simulink model "MR_CIGRE_CONVENCIONAL"  (R2017b)
settings: Solver=ode23tb  StartTime=0.0  StopTime=t_sim  RelTol=1e-4
values from neighbouring files (symbols this model uses):
  BAT1_CONT = 0    [Dados_MR_CIGRE_convencional.m]
  BAT2_CONT = 0    [Dados_MR_CIGRE_convencional.m]
  cont_fre = 1    [Dados_de_Sec.m]
  cont_ten = 1    [Dados_de_Sec.m]
  f0 = 50    [Dados_MR_CIGRE_convencional.m]
  Kie = 10    [Dados_de_Sec.m]
  Kiw = 2.5    [Dados_de_Sec.m]
  Kpe = 0.1    [Dados_de_Sec.m]
  Kpw = 0.23    [Dados_de_Sec.m]
  P_Solar1 = 21e3    (= 21000)    [Dados_MR_CIGRE_convencional.m]
  P_Solar2 = 21e3    (= 21000)    [Dados_MR_CIGRE_convencional.m]
  PQ_ref_time_bat1 = t_estab    (= 1)    [Dados_MR_CIGRE_convencional.m]
  Pref_Bat1 = 0*1e3    (= 0)    [Dados_MR_CIGRE_convencional.m]
  Qref_Bat1 = 0*1e3    (= 0)    [Dados_MR_CIGRE_convencional.m]
  Qref_Solar = 0    [Automatico_XXX.m]    (also in Dados_MR_CIGRE_convencional.m)
  Sb_Bat1 = 45e3    (= 45000)    [Dados_MR_CIGRE_convencional.m]
  Sb_sol1 = 20e3    (= 20000)    [Dados_MR_CIGRE_convencional.m]
  Sb_sol2 = 20e3    (= 20000)    [Dados_MR_CIGRE_convencional.m]
  t_atraso = 0    [Dados_MR_CIGRE_convencional.m]
  TDR1 = 80    [Dados_de_Cargas.m]
  TDR11 = 80    [Dados_de_Cargas.m]
  TDR15 = 80    [Dados_de_Cargas.m]
  TDR16 = 80    [Dados_de_Cargas.m]
  TDR17 = 80    [Dados_de_Cargas.m]
  TDR18 = 80    [Dados_de_Cargas.m]
  tilha = 0.6    [Dados_MR_CIGRE_convencional.m]
  TLR11 = 60    [Dados_de_Cargas.m]
  TLR15 = 3.5    [Dados_de_Cargas.m]
  TLR16 = 6    [Dados_de_Cargas.m]
  TLR17 = 60    [Dados_de_Cargas.m]
  TLR18 = 60    [Dados_de_Cargas.m]
  tsinc = 6    [Dados_MR_CIGRE_convencional.m]
  vref1 = 1    [Dados_de_Sec.m]
  Vref_sec = 1    [Dados_de_Sec.m]
  Vs1 = 20000    [Dados_MR_CIGRE_convencional.m]
  Vs2 = 400    [Dados_MR_CIGRE_convencional.m]
  w0 = 2*pi*f0    (= 314.159265359)    [Dados_MR_CIGRE_convencional.m]
  wref_sec = 1    [Dados_de_Sec.m]
undefined symbols (not defined in the file or in its folder): Cdc, Cdc_Bat1, Cf, Cf_Bat1, I_max_Bat1, Imax_solar1, Imax_solar2, Is_bat1, K_iff_Bat1, Kcij, Ki_Bat1, Ki_interm, Kp_Bat1, Kp_cp, Kp_cr, Kp_interm, Kv_Bat1, Kvi_DC, Kvp_DC, L, L_10_18, L_12_13, L_13_14, L_14_15, L_1_2, L_2_3, L_3_11, L_3_4, L_4_12, L_4_5, L_5_6, L_6_16, L_6_7, L_7_8, L_8_9, L_9_10, L_9_17, L_Bat1, L_Bat2, L_Virt_Bat1, L_Virt_Bat2, LC_Bat2, Lfsj, LPF_Ci_Bat1, LPF_Ci_Bat2, LPF_Cv_Bat1, LPF_P_Bat1, LPF_P_Interm, LPF_Q_Bat1, LPF_Vdc, m_Bat1, n_Bat1, PQ_ref_taxavar_bat1, R, R_10_18, R_12_13, R_13_14, R_14_15, R_1_2, R_2_3 ... (+27)
libraries: powerlib x158, powerlib_meascontrol x59, re_lib x2, simulink x1
(part 2 of 4)

== system MR_CIGRE_CONVENCIONAL/R11 ==
  1/Ib : Gain  Gain=(1)/(sqrt(2))
  1/Vb : Gain  Gain=sqrt(3)/(1*sqrt(2))
  BCarga : powerlib/Measurements/Three-Phase V-I Measurement  VoltageMeasurement=phase-to-ground  SetLabelV=off  LabelV=Vabc_B2  Vpu=off  VpuLL=off  CurrentMeasurement=yes  SetLabelI=off  LabelI=Iabc_B120  Ipu=off  Pbase=100e6  Vbase=Vs2  OutputType=Complex  PhasorSimulation=on  PSBequivalent=0
  CCV1 : powerlib/Elements/Three-Phase Breaker  InitialState=open  SwitchA=on  SwitchB=on  SwitchC=on  SwitchTimes=[TLR11 TDR11]  External=off  BreakerResistance=0.01  SnubberResistance=1e5  SnubberCapacitance=inf  Measurements=None
      settings: AttributesFormatString=\n
  Carga Fixa : powerlib/Elements/Three-Phase Series RLC Load  LConnTagsString=A|B|C  Configuration=Y (grounded)  NominalVoltage=Vs2  Vabc=[1e3 1e3 1e3]  Vabcp=[1e3 1e3 1e3]  NominalFrequency=f0  UnbalancedPower=off  ActivePower=PLoadR11  InductivePower=QLoadR11  CapacitivePower=0  Pabc=[10e3 9e3 11e3]  QLabc=[100 90 110]  QCabc=[100 90 110]  Pabcp=[10e3 9e3 11e3]  QLabcp=[100 90 110]  QCabcp=[100 90 110]  Measurements=None  LoadType=constant Z
  Carga Variável : powerlib/Elements/Three-Phase Series RLC Load  LConnTagsString=A|B|C  Configuration=Y (grounded)  NominalVoltage=Vs2  Vabc=[1e3 1e3 1e3]  Vabcp=[1e3 1e3 1e3]  NominalFrequency=f0  UnbalancedPower=off  ActivePower=P_var_loadR11  InductivePower=Q_var_loadR11  CapacitivePower=0  Pabc=[10e3 9e3 11e3]  QLabc=[100 90 110]  QCabc=[100 90 110]  Pabcp=[10e3 9e3 11e3]  QLabcp=[100 90 110]  QCabcp=[100 90 110]  Measurements=None  LoadType=constant Z
  Dados_C1 : ToWorkspace  VariableName=R11  SaveFormat=Structure With Time  SampleTime=-1
  Ip : powerlib_meascontrol/Measurements/Sequence Analyzer  Freq=f0  n=1  seq=Positive  InInit=[1, 0]  Ts=0
      settings: SourceProductName=Simscape Power Systems  SourceProductBaseCode=PS
  Mux9 : Mux
  Power : powerlib_meascontrol/Measurements/Power (Positive-Sequence)  Freq=f0  Vinit=[0, 0]  Iinit=[0, 0]  Ts=0
      settings: SourceProductName=Simscape Power Systems  SourceProductBaseCode=PS
  Reshape : Reshape  OutputDimensions=[1,7]
  Vp : powerlib_meascontrol/Measurements/Sequence Analyzer  Freq=f0  n=1  seq=Positive  InInit=[1, 0]  Ts=0
      settings: SourceProductName=Simscape Power Systems  SourceProductBaseCode=PS
  fa : PMIOPort  Port=1  Side=Left
  fb : PMIOPort  Port=2  Side=Left
  fc : PMIOPort  Port=3  Side=Left
  P : Outport
  V : Outport  Port=2
  Q : Outport  Port=3
  I : Outport  Port=4
  wires:
  BCarga/1 -> Power/1, Vp/1
  Mux9/1 -> Reshape/1
  BCarga/2 -> Power/2, Ip/1
  Power/1 -> Mux9/1, P/1
  1/Vb/1 -> V/1, Mux9/2
  1/Ib/1 -> I/1, Mux9/4
  Vp/1 -> 1/Vb/1
  Ip/1 -> 1/Ib/1
  Power/2 -> Q/1, Mux9/3
  Reshape/1 -> Dados_C1/1
  connections:
  BCarga/LConn3 -- fc/RConn1
  BCarga/LConn2 -- fb/RConn1
  BCarga/LConn1 -- fa/RConn1
  BCarga/RConn3 -- CCV1/RConn3 -- Carga Fixa/LConn3
  BCarga/RConn1 -- CCV1/RConn1 -- Carga Fixa/LConn1
  BCarga/RConn2 -- CCV1/RConn2 -- Carga Fixa/LConn2
  CCV1/LConn1 -- Carga Variável/LConn1
  CCV1/LConn3 -- Carga Variável/LConn3
  CCV1/LConn2 -- Carga Variável/LConn2

== system MR_CIGRE_CONVENCIONAL/R12_R13 ==
  1 : powerlib/Elements/Series RLC Branch  LConnTagsString=__new0  RConnTagsString=__new0  BranchType=RL  Resistance=R_12_13  Inductance=L_12_13  SetiL0=off  InitialCurrent=0  Capacitance=1e-6  Setx0=off  InitialVoltage=0  Measurements=None
  2 : powerlib/Elements/Series RLC Branch  LConnTagsString=__new0  RConnTagsString=__new0  BranchType=RL  Resistance=R_12_13  Inductance=L_12_13  SetiL0=off  InitialCurrent=0  Capacitance=1e-6  Setx0=off  InitialVoltage=0  Measurements=None
  3 : powerlib/Elements/Series RLC Branch  LConnTagsString=__new0  RConnTagsString=__new0  BranchType=RL  Resistance=R_12_13  Inductance=L_12_13  SetiL0=off  InitialCurrent=0  Capacitance=1e-6  Setx0=off  InitialVoltage=0  Measurements=None
  A : PMIOPort  Port=1  Side=Left
  a : PMIOPort  Port=2  Side=Right
  B : PMIOPort  Port=3  Side=Left
  b : PMIOPort  Port=4  Side=Right
  C : PMIOPort  Port=5  Side=Left
  c : PMIOPort  Port=6  Side=Right
  connections:
  1/LConn1 -- A/RConn1
  2/LConn1 -- B/RConn1
  3/LConn1 -- C/RConn1
  1/RConn1 -- a/RConn1
  2/RConn1 -- b/RConn1
  3/RConn1 -- c/RConn1

== system MR_CIGRE_CONVENCIONAL/R13_R14 ==
  1 : powerlib/Elements/Series RLC Branch  LConnTagsString=__new0  RConnTagsString=__new0  BranchType=RL  Resistance=R_13_14  Inductance=L_13_14  SetiL0=off  InitialCurrent=0  Capacitance=1e-6  Setx0=off  InitialVoltage=0  Measurements=None
  2 : powerlib/Elements/Series RLC Branch  LConnTagsString=__new0  RConnTagsString=__new0  BranchType=RL  Resistance=R_13_14  Inductance=L_13_14  SetiL0=off  InitialCurrent=0  Capacitance=1e-6  Setx0=off  InitialVoltage=0  Measurements=None
  3 : powerlib/Elements/Series RLC Branch  LConnTagsString=__new0  RConnTagsString=__new0  BranchType=RL  Resistance=R_13_14  Inductance=L_13_14  SetiL0=off  InitialCurrent=0  Capacitance=1e-6  Setx0=off  InitialVoltage=0  Measurements=None
  A : PMIOPort  Port=1  Side=Left
  a : PMIOPort  Port=2  Side=Right
  B : PMIOPort  Port=3  Side=Left
  b : PMIOPort  Port=4  Side=Right
  C : PMIOPort  Port=5  Side=Left
  c : PMIOPort  Port=6  Side=Right
  connections:
  1/LConn1 -- A/RConn1
  2/LConn1 -- B/RConn1
  3/LConn1 -- C/RConn1
  1/RConn1 -- a/RConn1
  2/RConn1 -- b/RConn1
  3/RConn1 -- c/RConn1

== system MR_CIGRE_CONVENCIONAL/R14_R15 ==
  1 : powerlib/Elements/Series RLC Branch  LConnTagsString=__new0  RConnTagsString=__new0  BranchType=RL  Resistance=R_14_15  Inductance=L_14_15  SetiL0=off  InitialCurrent=0  Capacitance=1e-6  Setx0=off  InitialVoltage=0  Measurements=None
  2 : powerlib/Elements/Series RLC Branch  LConnTagsString=__new0  RConnTagsString=__new0  BranchType=RL  Resistance=R_14_15  Inductance=L_14_15  SetiL0=off  InitialCurrent=0  Capacitance=1e-6  Setx0=off  InitialVoltage=0  Measurements=None
  3 : powerlib/Elements/Series RLC Branch  LConnTagsString=__new0  RConnTagsString=__new0  BranchType=RL  Resistance=R_14_15  Inductance=L_14_15  SetiL0=off  InitialCurrent=0  Capacitance=1e-6  Setx0=off  InitialVoltage=0  Measurements=None
  A : PMIOPort  Port=1  Side=Left
  a : PMIOPort  Port=2  Side=Right
  B : PMIOPort  Port=3  Side=Left
  b : PMIOPort  Port=4  Side=Right
  C : PMIOPort  Port=5  Side=Left
  c : PMIOPort  Port=6  Side=Right
  connections:
  1/LConn1 -- A/RConn1
  2/LConn1 -- B/RConn1
  3/LConn1 -- C/RConn1
  1/RConn1 -- a/RConn1
  2/RConn1 -- b/RConn1
  3/RConn1 -- c/RConn1

== system MR_CIGRE_CONVENCIONAL/R15 ==
  1/Ib : Gain  Gain=(1)/(sqrt(2))
  1/Vb : Gain  Gain=sqrt(3)/(1*sqrt(2))
  BCarga : powerlib/Measurements/Three-Phase V-I Measurement  VoltageMeasurement=phase-to-ground  SetLabelV=off  LabelV=Vabc_B2  Vpu=off  VpuLL=off  CurrentMeasurement=yes  SetLabelI=off  LabelI=Iabc_B120  Ipu=off  Pbase=100e6  Vbase=Vs2  OutputType=Complex  PhasorSimulation=on  PSBequivalent=0
  CCV : powerlib/Elements/Three-Phase Breaker  InitialState=open  SwitchA=on  SwitchB=on  SwitchC=on  SwitchTimes=[TLR15 TDR15]  External=off  BreakerResistance=0.01  SnubberResistance=1e5  SnubberCapacitance=inf  Measurements=None
      settings: AttributesFormatString=\n
  Carga Fixa : powerlib/Elements/Three-Phase Series RLC Load  LConnTagsString=A|B|C  Configuration=Y (grounded)  NominalVoltage=Vs2  Vabc=[1e3 1e3 1e3]  Vabcp=[1e3 1e3 1e3]  NominalFrequency=f0  UnbalancedPower=off  ActivePower=PLoadR15  InductivePower=QLoadR15  CapacitivePower=0  Pabc=[10e3 9e3 11e3]  QLabc=[100 90 110]  QCabc=[100 90 110]  Pabcp=[10e3 9e3 11e3]  QLabcp=[100 90 110]  QCabcp=[100 90 110]  Measurements=None  LoadType=constant Z
  Carga Variável : powerlib/Elements/Three-Phase Series RLC Load  LConnTagsString=A|B|C  Configuration=Y (grounded)  NominalVoltage=Vs2  Vabc=[1e3 1e3 1e3]  Vabcp=[1e3 1e3 1e3]  NominalFrequency=f0  UnbalancedPower=off  ActivePower=P_var_loadR15  InductivePower=Q_var_loadR15  CapacitivePower=0  Pabc=[10e3 9e3 11e3]  QLabc=[100 90 110]  QCabc=[100 90 110]  Pabcp=[10e3 9e3 11e3]  QLabcp=[100 90 110]  QCabcp=[100 90 110]  Measurements=None  LoadType=constant Z
  Dados_C1 : ToWorkspace  VariableName=R15  SaveFormat=Structure With Time  SampleTime=-1
  Ip : powerlib_meascontrol/Measurements/Sequence Analyzer  Freq=f0  n=1  seq=Positive  InInit=[1, 0]  Ts=0
      settings: SourceProductName=Simscape Power Systems  SourceProductBaseCode=PS
  Mux9 : Mux
  Power : powerlib_meascontrol/Measurements/Power (Positive-Sequence)  Freq=f0  Vinit=[0, 0]  Iinit=[0, 0]  Ts=0
      settings: SourceProductName=Simscape Power Systems  SourceProductBaseCode=PS
  Reshape : Reshape  OutputDimensions=[1,7]
  Vp : powerlib_meascontrol/Measurements/Sequence Analyzer  Freq=f0  n=1  seq=Positive  InInit=[1, 0]  Ts=0
      settings: SourceProductName=Simscape Power Systems  SourceProductBaseCode=PS
  fa : PMIOPort  Port=1  Side=Left
  fb : PMIOPort  Port=2  Side=Left
  fc : PMIOPort  Port=3  Side=Left
  P : Outport
  V : Outport  Port=2
  Q : Outport  Port=3
  I : Outport  Port=4
  wires:
  Mux9/1 -> Reshape/1
  BCarga/2 -> Power/2, Ip/1
  1/Ib/1 -> I/1, Mux9/4
  Ip/1 -> 1/Ib/1
  1/Vb/1 -> V/1, Mux9/2
  Vp/1 -> 1/Vb/1
  BCarga/1 -> Power/1, Vp/1
  Power/2 -> Q/1, Mux9/3
  Power/1 -> Mux9/1, P/1
  Reshape/1 -> Dados_C1/1
  connections:
  BCarga/LConn3 -- fc/RConn1
  BCarga/LConn2 -- fb/RConn1
  BCarga/LConn1 -- fa/RConn1
  BCarga/RConn3 -- Carga Fixa/LConn3 -- CCV/RConn3
  BCarga/RConn1 -- Carga Fixa/LConn1 -- CCV/RConn1
  BCarga/RConn2 -- Carga Fixa/LConn2 -- CCV/RConn2
  CCV/LConn1 -- Carga Variável/LConn1
  CCV/LConn3 -- Carga Variável/LConn3
  CCV/LConn2 -- Carga Variável/LConn2

== system MR_CIGRE_CONVENCIONAL/R16 ==
  1/Ib : Gain  Gain=(1)/(sqrt(2))
  1/Vb : Gain  Gain=sqrt(3)/(1*sqrt(2))
  BCarga : powerlib/Measurements/Three-Phase V-I Measurement  VoltageMeasurement=phase-to-ground  SetLabelV=off  LabelV=Vabc_B2  Vpu=off  VpuLL=off  CurrentMeasurement=yes  SetLabelI=off  LabelI=Iabc_B120  Ipu=off  Pbase=100e6  Vbase=Vs2  OutputType=Complex  PhasorSimulation=on  PSBequivalent=0
  CCV : powerlib/Elements/Three-Phase Breaker  InitialState=open  SwitchA=on  SwitchB=on  SwitchC=on  SwitchTimes=[TLR16 TDR16]  External=off  BreakerResistance=0.01  SnubberResistance=1e5  SnubberCapacitance=inf  Measurements=None
      settings: AttributesFormatString=\n
  Carga Fixa : powerlib/Elements/Three-Phase Series RLC Load  LConnTagsString=A|B|C  Configuration=Y (grounded)  NominalVoltage=Vs2  Vabc=[1e3 1e3 1e3]  Vabcp=[1e3 1e3 1e3]  NominalFrequency=f0  UnbalancedPower=off  ActivePower=PLoadR16  InductivePower=QLoadR16  CapacitivePower=0  Pabc=[10e3 9e3 11e3]  QLabc=[100 90 110]  QCabc=[100 90 110]  Pabcp=[10e3 9e3 11e3]  QLabcp=[100 90 110]  QCabcp=[100 90 110]  Measurements=None  LoadType=constant Z
  Carga Variável : powerlib/Elements/Three-Phase Series RLC Load  LConnTagsString=A|B|C  Configuration=Y (grounded)  NominalVoltage=Vs2  Vabc=[1e3 1e3 1e3]  Vabcp=[1e3 1e3 1e3]  NominalFrequency=f0  UnbalancedPower=off  ActivePower=P_var_loadR16  InductivePower=Q_var_loadR16  CapacitivePower=0  Pabc=[10e3 9e3 11e3]  QLabc=[100 90 110]  QCabc=[100 90 110]  Pabcp=[10e3 9e3 11e3]  QLabcp=[100 90 110]  QCabcp=[100 90 110]  Measurements=None  LoadType=constant Z
  Dados_C1 : ToWorkspace  VariableName=R16  SaveFormat=Structure With Time  SampleTime=-1
  Ip : powerlib_meascontrol/Measurements/Sequence Analyzer  Freq=f0  n=1  seq=Positive  InInit=[1, 0]  Ts=0
      settings: SourceProductName=Simscape Power Systems  SourceProductBaseCode=PS
  Mux9 : Mux
  Power : powerlib_meascontrol/Measurements/Power (Positive-Sequence)  Freq=f0  Vinit=[0, 0]  Iinit=[0, 0]  Ts=0
      settings: SourceProductName=Simscape Power Systems  SourceProductBaseCode=PS
  Reshape : Reshape  OutputDimensions=[1,7]
  Vp : powerlib_meascontrol/Measurements/Sequence Analyzer  Freq=f0  n=1  seq=Positive  InInit=[1, 0]  Ts=0
      settings: SourceProductName=Simscape Power Systems  SourceProductBaseCode=PS
  fa : PMIOPort  Port=1  Side=Left
  fb : PMIOPort  Port=2  Side=Left
  fc : PMIOPort  Port=3  Side=Left
  P : Outport
  V : Outport  Port=2
  Q : Outport  Port=3
  I : Outport  Port=4
  wires:
  Mux9/1 -> Reshape/1
  BCarga/2 -> Power/2, Ip/1
  1/Ib/1 -> Mux9/4, I/1
  Ip/1 -> 1/Ib/1
  1/Vb/1 -> V/1, Mux9/2
  Vp/1 -> 1/Vb/1
  BCarga/1 -> Power/1, Vp/1
  Power/2 -> Q/1, Mux9/3
  Power/1 -> Mux9/1, P/1
  Reshape/1 -> Dados_C1/1
  connections:
  BCarga/LConn3 -- fc/RConn1
  BCarga/LConn2 -- fb/RConn1
  BCarga/LConn1 -- fa/RConn1
  BCarga/RConn3 -- CCV/RConn3 -- Carga Fixa/LConn3
  BCarga/RConn1 -- CCV/RConn1 -- Carga Fixa/LConn1
  BCarga/RConn2 -- CCV/RConn2 -- Carga Fixa/LConn2
  CCV/LConn1 -- Carga Variável/LConn1
  CCV/LConn3 -- Carga Variável/LConn3
  CCV/LConn2 -- Carga Variável/LConn2

== system MR_CIGRE_CONVENCIONAL/R17 ==
  1/Ib : Gain  Gain=(1)/(sqrt(2))
  1/Vb : Gain  Gain=sqrt(3)/(1*sqrt(2))
  BCarga : powerlib/Measurements/Three-Phase V-I Measurement  VoltageMeasurement=phase-to-ground  SetLabelV=off  LabelV=Vabc_B2  Vpu=off  VpuLL=off  CurrentMeasurement=yes  SetLabelI=off  LabelI=Iabc_B120  Ipu=off  Pbase=100e6  Vbase=Vs2  OutputType=Complex  PhasorSimulation=on  PSBequivalent=0
  CCV1 : powerlib/Elements/Three-Phase Breaker  InitialState=open  SwitchA=on  SwitchB=on  SwitchC=on  SwitchTimes=[TLR17 TDR17]  External=off  BreakerResistance=0.01  SnubberResistance=1e5  SnubberCapacitance=inf  Measurements=None
      settings: AttributesFormatString=\n
  Carga Fixa : powerlib/Elements/Three-Phase Series RLC Load  LConnTagsString=A|B|C  Configuration=Y (grounded)  NominalVoltage=Vs2  Vabc=[1e3 1e3 1e3]  Vabcp=[1e3 1e3 1e3]  NominalFrequency=f0  UnbalancedPower=off  ActivePower=PLoadR17  InductivePower=QLoadR17  CapacitivePower=0  Pabc=[10e3 9e3 11e3]  QLabc=[100 90 110]  QCabc=[100 90 110]  Pabcp=[10e3 9e3 11e3]  QLabcp=[100 90 110]  QCabcp=[100 90 110]  Measurements=None  LoadType=constant Z
  Carga Variável : powerlib/Elements/Three-Phase Series RLC Load  LConnTagsString=A|B|C  Configuration=Y (grounded)  NominalVoltage=Vs2  Vabc=[1e3 1e3 1e3]  Vabcp=[1e3 1e3 1e3]  NominalFrequency=f0  UnbalancedPower=off  ActivePower=P_var_loadR17  InductivePower=Q_var_loadR17  CapacitivePower=0  Pabc=[10e3 9e3 11e3]  QLabc=[100 90 110]  QCabc=[100 90 110]  Pabcp=[10e3 9e3 11e3]  QLabcp=[100 90 110]  QCabcp=[100 90 110]  Measurements=None  LoadType=constant Z
  Dados_C1 : ToWorkspace  VariableName=R17  SaveFormat=Structure With Time  SampleTime=-1
  Ip : powerlib_meascontrol/Measurements/Sequence Analyzer  Freq=f0  n=1  seq=Positive  InInit=[1, 0]  Ts=0
      settings: SourceProductName=Simscape Power Systems  SourceProductBaseCode=PS
  Mux9 : Mux
  Power : powerlib_meascontrol/Measurements/Power (Positive-Sequence)  Freq=f0  Vinit=[0, 0]  Iinit=[0, 0]  Ts=0
      settings: SourceProductName=Simscape Power Systems  SourceProductBaseCode=PS
  Reshape : Reshape  OutputDimensions=[1,7]
  Vp : powerlib_meascontrol/Measurements/Sequence Analyzer  Freq=f0  n=1  seq=Positive  InInit=[1, 0]  Ts=0
      settings: SourceProductName=Simscape Power Systems  SourceProductBaseCode=PS
  fa : PMIOPort  Port=1  Side=Left
  fb : PMIOPort  Port=2  Side=Left
  fc : PMIOPort  Port=3  Side=Left
  P : Outport
  V : Outport  Port=2
  Q : Outport  Port=3
  I : Outport  Port=4
  wires:
  Mux9/1 -> Reshape/1
  BCarga/2 -> Power/2, Ip/1
  1/Ib/1 -> I/1, Mux9/4
  Ip/1 -> 1/Ib/1
  1/Vb/1 -> Mux9/2, V/1
  Vp/1 -> 1/Vb/1
  BCarga/1 -> Power/1, Vp/1
  Power/2 -> Q/1, Mux9/3
  Power/1 -> Mux9/1, P/1
  Reshape/1 -> Dados_C1/1
  connections:
  BCarga/LConn3 -- fc/RConn1
  BCarga/LConn2 -- fb/RConn1
  BCarga/LConn1 -- fa/RConn1
  BCarga/RConn3 -- CCV1/RConn3 -- Carga Fixa/LConn3
  BCarga/RConn1 -- CCV1/RConn1 -- Carga Fixa/LConn1
  BCarga/RConn2 -- CCV1/RConn2 -- Carga Fixa/LConn2
  CCV1/LConn1 -- Carga Variável/LConn1
  CCV1/LConn3 -- Carga Variável/LConn3
  CCV1/LConn2 -- Carga Variável/LConn2

== system MR_CIGRE_CONVENCIONAL/R18 ==
  1/Ib : Gain  Gain=(1)/(sqrt(2))
  1/Vb : Gain  Gain=sqrt(3)/(1*sqrt(2))
  BCarga : powerlib/Measurements/Three-Phase V-I Measurement  VoltageMeasurement=phase-to-ground  SetLabelV=off  LabelV=Vabc_B2  Vpu=off  VpuLL=off  CurrentMeasurement=yes  SetLabelI=off  LabelI=Iabc_B120  Ipu=off  Pbase=100e6  Vbase=Vs2  OutputType=Complex  PhasorSimulation=on  PSBequivalent=0
  CCV : powerlib/Elements/Three-Phase Breaker  InitialState=open  SwitchA=on  SwitchB=on  SwitchC=on  SwitchTimes=[TLR18 TDR18]  External=off  BreakerResistance=0.01  SnubberResistance=1e5  SnubberCapacitance=inf  Measurements=None
      settings: AttributesFormatString=\n
  Carga Fixa : powerlib/Elements/Three-Phase Series RLC Load  LConnTagsString=A|B|C  Configuration=Y (grounded)  NominalVoltage=Vs2  Vabc=[1e3 1e3 1e3]  Vabcp=[1e3 1e3 1e3]  NominalFrequency=f0  UnbalancedPower=off  ActivePower=PLoadR18  InductivePower=QLoadR18  CapacitivePower=0  Pabc=[10e3 9e3 11e3]  QLabc=[100 90 110]  QCabc=[100 90 110]  Pabcp=[10e3 9e3 11e3]  QLabcp=[100 90 110]  QCabcp=[100 90 110]  Measurements=None  LoadType=constant Z
  Carga Variável : powerlib/Elements/Three-Phase Series RLC Load  LConnTagsString=A|B|C  Configuration=Y (grounded)  NominalVoltage=Vs2  Vabc=[1e3 1e3 1e3]  Vabcp=[1e3 1e3 1e3]  NominalFrequency=f0  UnbalancedPower=off  ActivePower=P_var_loadR18  InductivePower=Q_var_loadR18  CapacitivePower=0  Pabc=[10e3 9e3 11e3]  QLabc=[100 90 110]  QCabc=[100 90 110]  Pabcp=[10e3 9e3 11e3]  QLabcp=[100 90 110]  QCabcp=[100 90 110]  Measurements=None  LoadType=constant Z
  Dados_C1 : ToWorkspace  VariableName=R18  SaveFormat=Structure With Time  SampleTime=-1
  Ip : powerlib_meascontrol/Measurements/Sequence Analyzer  Freq=f0  n=1  seq=Positive  InInit=[1, 0]  Ts=0
      settings: SourceProductName=Simscape Power Systems  SourceProductBaseCode=PS
  Mux9 : Mux
  Power : powerlib_meascontrol/Measurements/Power (Positive-Sequence)  Freq=f0  Vinit=[0, 0]  Iinit=[0, 0]  Ts=0
      settings: SourceProductName=Simscape Power Systems  SourceProductBaseCode=PS
  Reshape : Reshape  OutputDimensions=[1,7]
  Vp : powerlib_meascontrol/Measurements/Sequence Analyzer  Freq=f0  n=1  seq=Positive  InInit=[1, 0]  Ts=0
      settings: SourceProductName=Simscape Power Systems  SourceProductBaseCode=PS
  fa : PMIOPort  Port=1  Side=Left
  fb : PMIOPort  Port=2  Side=Left
  fc : PMIOPort  Port=3  Side=Left
  P : Outport
  V : Outport  Port=2
  Q : Outport  Port=3
  I : Outport  Port=4
  wires:
  Mux9/1 -> Reshape/1
  BCarga/2 -> Power/2, Ip/1
  1/Ib/1 -> Mux9/4, I/1
  Ip/1 -> 1/Ib/1
  1/Vb/1 -> Mux9/2, V/1
  Vp/1 -> 1/Vb/1
  BCarga/1 -> Power/1, Vp/1
  Power/2 -> Q/1, Mux9/3
  Power/1 -> Mux9/1, P/1
  Reshape/1 -> Dados_C1/1
  connections:
  BCarga/LConn3 -- fc/RConn1
  BCarga/LConn2 -- fb/RConn1
  BCarga/LConn1 -- fa/RConn1
  BCarga/RConn3 -- CCV/RConn3 -- Carga Fixa/LConn3
  BCarga/RConn1 -- CCV/RConn1 -- Carga Fixa/LConn1
  BCarga/RConn2 -- CCV/RConn2 -- Carga Fixa/LConn2
  CCV/LConn1 -- Carga Variável/LConn1
  CCV/LConn3 -- Carga Variável/LConn3
  CCV/LConn2 -- Carga Variável/LConn2

== system MR_CIGRE_CONVENCIONAL/R2-R3 ==
  1 : powerlib/Elements/Series RLC Branch  LConnTagsString=__new0  RConnTagsString=__new0  BranchType=RL  Resistance=R_2_3  Inductance=L_2_3  SetiL0=off  InitialCurrent=0  Capacitance=1e-6  Setx0=off  InitialVoltage=0  Measurements=None
  2 : powerlib/Elements/Series RLC Branch  LConnTagsString=__new0  RConnTagsString=__new0  BranchType=RL  Resistance=R_2_3  Inductance=L_2_3  SetiL0=off  InitialCurrent=0  Capacitance=1e-6  Setx0=off  InitialVoltage=0  Measurements=None
  3 : powerlib/Elements/Series RLC Branch  LConnTagsString=__new0  RConnTagsString=__new0  BranchType=RL  Resistance=R_2_3  Inductance=L_2_3  SetiL0=off  InitialCurrent=0  Capacitance=1e-6  Setx0=off  InitialVoltage=0  Measurements=None
  A : PMIOPort  Port=1  Side=Left
  a : PMIOPort  Port=2  Side=Right
  B : PMIOPort  Port=3  Side=Left
  b : PMIOPort  Port=4  Side=Right
  C : PMIOPort  Port=5  Side=Left
  c : PMIOPort  Port=6  Side=Right
  connections:
  1/LConn1 -- A/RConn1
  2/LConn1 -- B/RConn1
  3/LConn1 -- C/RConn1
  1/RConn1 -- a/RConn1
  2/RConn1 -- b/RConn1
  3/RConn1 -- c/RConn1

== system MR_CIGRE_CONVENCIONAL/R3_R11 ==
  1 : powerlib/Elements/Series RLC Branch  LConnTagsString=__new0  RConnTagsString=__new0  BranchType=RL  Resistance=R_3_11  Inductance=L_3_11  SetiL0=off  InitialCurrent=0  Capacitance=1e-6  Setx0=off  InitialVoltage=0  Measurements=None
  2 : powerlib/Elements/Series RLC Branch  LConnTagsString=__new0  RConnTagsString=__new0  BranchType=RL  Resistance=R_3_11  Inductance=L_3_11  SetiL0=off  InitialCurrent=0  Capacitance=1e-6  Setx0=off  InitialVoltage=0  Measurements=None
  3 : powerlib/Elements/Series RLC Branch  LConnTagsString=__new0  RConnTagsString=__new0  BranchType=RL  Resistance=R_3_11  Inductance=L_3_11  SetiL0=off  InitialCurrent=0  Capacitance=1e-6  Setx0=off  InitialVoltage=0  Measurements=None
  A : PMIOPort  Port=1  Side=Left
  a : PMIOPort  Port=2  Side=Right
  B : PMIOPort  Port=3  Side=Left
  b : PMIOPort  Port=4  Side=Right
  C : PMIOPort  Port=5  Side=Left
  c : PMIOPort  Port=6  Side=Right
  connections:
  1/LConn1 -- A/RConn1
  2/LConn1 -- B/RConn1
  3/LConn1 -- C/RConn1
  1/RConn1 -- a/RConn1
  2/RConn1 -- b/RConn1
  3/RConn1 -- c/RConn1

== system MR_CIGRE_CONVENCIONAL/R3_R4 ==
  1 : powerlib/Elements/Series RLC Branch  LConnTagsString=__new0  RConnTagsString=__new0  BranchType=RL  Resistance=R_3_4  Inductance=L_3_4  SetiL0=off  InitialCurrent=0  Capacitance=1e-6  Setx0=off  InitialVoltage=0  Measurements=None
  2 : powerlib/Elements/Series RLC Branch  LConnTagsString=__new0  RConnTagsString=__new0  BranchType=RL  Resistance=R_3_4  Inductance=L_3_4  SetiL0=off  InitialCurrent=0  Capacitance=1e-6  Setx0=off  InitialVoltage=0  Measurements=None
  3 : powerlib/Elements/Series RLC Branch  LConnTagsString=__new0  RConnTagsString=__new0  BranchType=RL  Resistance=R_3_4  Inductance=L_3_4  SetiL0=off  InitialCurrent=0  Capacitance=1e-6  Setx0=off  InitialVoltage=0  Measurements=None
  A : PMIOPort  Port=1  Side=Left
  a : PMIOPort  Port=2  Side=Right
  B : PMIOPort  Port=3  Side=Left
  b : PMIOPort  Port=4  Side=Right
  C : PMIOPort  Port=5  Side=Left
  c : PMIOPort  Port=6  Side=Right
  connections:
  1/LConn1 -- A/RConn1
  2/LConn1 -- B/RConn1
  3/LConn1 -- C/RConn1
  1/RConn1 -- a/RConn1
  2/RConn1 -- b/RConn1
  3/RConn1 -- c/RConn1

== system MR_CIGRE_CONVENCIONAL/R4_R12 ==
  1 : powerlib/Elements/Series RLC Branch  LConnTagsString=__new0  RConnTagsString=__new0  BranchType=RL  Resistance=R_4_12  Inductance=L_4_12  SetiL0=off  InitialCurrent=0  Capacitance=1e-6  Setx0=off  InitialVoltage=0  Measurements=None
  2 : powerlib/Elements/Series RLC Branch  LConnTagsString=__new0  RConnTagsString=__new0  BranchType=RL  Resistance=R_4_12  Inductance=L_4_12  SetiL0=off  InitialCurrent=0  Capacitance=1e-6  Setx0=off  InitialVoltage=0  Measurements=None
  3 : powerlib/Elements/Series RLC Branch  LConnTagsString=__new0  RConnTagsString=__new0  BranchType=RL  Resistance=R_4_12  Inductance=L_4_12  SetiL0=off  InitialCurrent=0  Capacitance=1e-6  Setx0=off  InitialVoltage=0  Measurements=None
  A : PMIOPort  Port=1  Side=Left
  a : PMIOPort  Port=2  Side=Right
  B : PMIOPort  Port=3  Side=Left
  b : PMIOPort  Port=4  Side=Right
  C : PMIOPort  Port=5  Side=Left
  c : PMIOPort  Port=6  Side=Right
  connections:
  1/LConn1 -- A/RConn1
  2/LConn1 -- B/RConn1
  3/LConn1 -- C/RConn1
  1/RConn1 -- a/RConn1
  2/RConn1 -- b/RConn1
  3/RConn1 -- c/RConn1

== system MR_CIGRE_CONVENCIONAL/R4_R5 ==
  1 : powerlib/Elements/Series RLC Branch  LConnTagsString=__new0  RConnTagsString=__new0  BranchType=RL  Resistance=R_4_5  Inductance=L_4_5  SetiL0=off  InitialCurrent=0  Capacitance=1e-6  Setx0=off  InitialVoltage=0  Measurements=None
  2 : powerlib/Elements/Series RLC Branch  LConnTagsString=__new0  RConnTagsString=__new0  BranchType=RL  Resistance=R_4_5  Inductance=L_4_5  SetiL0=off  InitialCurrent=0  Capacitance=1e-6  Setx0=off  InitialVoltage=0  Measurements=None
  3 : powerlib/Elements/Series RLC Branch  LConnTagsString=__new0  RConnTagsString=__new0  BranchType=RL  Resistance=R_4_5  Inductance=L_4_5  SetiL0=off  InitialCurrent=0  Capacitance=1e-6  Setx0=off  InitialVoltage=0  Measurements=None
  A : PMIOPort  Port=1  Side=Left
  a : PMIOPort  Port=2  Side=Right
  B : PMIOPort  Port=3  Side=Left
  b : PMIOPort  Port=4  Side=Right
  C : PMIOPort  Port=5  Side=Left
  c : PMIOPort  Port=6  Side=Right
  connections:
  1/LConn1 -- A/RConn1
  2/LConn1 -- B/RConn1
  3/LConn1 -- C/RConn1
  1/RConn1 -- a/RConn1
  2/RConn1 -- b/RConn1
  3/RConn1 -- c/RConn1

== system MR_CIGRE_CONVENCIONAL/R5_R6 ==
  1 : powerlib/Elements/Series RLC Branch  LConnTagsString=__new0  RConnTagsString=__new0  BranchType=RL  Resistance=R_5_6  Inductance=L_5_6  SetiL0=off  InitialCurrent=0  Capacitance=1e-6  Setx0=off  InitialVoltage=0  Measurements=None
  2 : powerlib/Elements/Series RLC Branch  LConnTagsString=__new0  RConnTagsString=__new0  BranchType=RL  Resistance=R_5_6  Inductance=L_5_6  SetiL0=off  InitialCurrent=0  Capacitance=1e-6  Setx0=off  InitialVoltage=0  Measurements=None
  3 : powerlib/Elements/Series RLC Branch  LConnTagsString=__new0  RConnTagsString=__new0  BranchType=RL  Resistance=R_5_6  Inductance=L_5_6  SetiL0=off  InitialCurrent=0  Capacitance=1e-6  Setx0=off  InitialVoltage=0  Measurements=None
  A : PMIOPort  Port=1  Side=Left
  a : PMIOPort  Port=2  Side=Right
  B : PMIOPort  Port=3  Side=Left
  b : PMIOPort  Port=4  Side=Right
  C : PMIOPort  Port=5  Side=Left
  c : PMIOPort  Port=6  Side=Right
  connections:
  1/LConn1 -- A/RConn1
  2/LConn1 -- B/RConn1
  3/LConn1 -- C/RConn1
  1/RConn1 -- a/RConn1
  2/RConn1 -- b/RConn1
  3/RConn1 -- c/RConn1

== system MR_CIGRE_CONVENCIONAL/R6_R16 ==
  1 : powerlib/Elements/Series RLC Branch  LConnTagsString=__new0  RConnTagsString=__new0  BranchType=RL  Resistance=R_6_16  Inductance=L_6_16  SetiL0=off  InitialCurrent=0  Capacitance=1e-6  Setx0=off  InitialVoltage=0  Measurements=None
  2 : powerlib/Elements/Series RLC Branch  LConnTagsString=__new0  RConnTagsString=__new0  BranchType=RL  Resistance=R_6_16  Inductance=L_6_16  SetiL0=off  InitialCurrent=0  Capacitance=1e-6  Setx0=off  InitialVoltage=0  Measurements=None
  3 : powerlib/Elements/Series RLC Branch  LConnTagsString=__new0  RConnTagsString=__new0  BranchType=RL  Resistance=R_6_16  Inductance=L_6_16  SetiL0=off  InitialCurrent=0  Capacitance=1e-6  Setx0=off  InitialVoltage=0  Measurements=None
  A : PMIOPort  Port=1  Side=Left
  a : PMIOPort  Port=2  Side=Right
  B : PMIOPort  Port=3  Side=Left
  b : PMIOPort  Port=4  Side=Right
  C : PMIOPort  Port=5  Side=Left
  c : PMIOPort  Port=6  Side=Right
  connections:
  1/LConn1 -- A/RConn1
  2/LConn1 -- B/RConn1
  3/LConn1 -- C/RConn1
  1/RConn1 -- a/RConn1
  2/RConn1 -- b/RConn1
  3/RConn1 -- c/RConn1

== system MR_CIGRE_CONVENCIONAL/R6_R7 ==
  1 : powerlib/Elements/Series RLC Branch  LConnTagsString=__new0  RConnTagsString=__new0  BranchType=RL  Resistance=R_6_7  Inductance=L_6_7  SetiL0=off  InitialCurrent=0  Capacitance=1e-6  Setx0=off  InitialVoltage=0  Measurements=None
  2 : powerlib/Elements/Series RLC Branch  LConnTagsString=__new0  RConnTagsString=__new0  BranchType=RL  Resistance=R_6_7  Inductance=L_6_7  SetiL0=off  InitialCurrent=0  Capacitance=1e-6  Setx0=off  InitialVoltage=0  Measurements=None
  3 : powerlib/Elements/Series RLC Branch  LConnTagsString=__new0  RConnTagsString=__new0  BranchType=RL  Resistance=R_6_7  Inductance=L_6_7  SetiL0=off  InitialCurrent=0  Capacitance=1e-6  Setx0=off  InitialVoltage=0  Measurements=None
  A : PMIOPort  Port=1  Side=Left
  a : PMIOPort  Port=2  Side=Right
  B : PMIOPort  Port=3  Side=Left
  b : PMIOPort  Port=4  Side=Right
  C : PMIOPort  Port=5  Side=Left
  c : PMIOPort  Port=6  Side=Right
  connections:
  1/LConn1 -- A/RConn1
  2/LConn1 -- B/RConn1
  3/LConn1 -- C/RConn1
  1/RConn1 -- a/RConn1
  2/RConn1 -- b/RConn1
  3/RConn1 -- c/RConn1

== system MR_CIGRE_CONVENCIONAL/R7_R8 ==
  1 : powerlib/Elements/Series RLC Branch  LConnTagsString=__new0  RConnTagsString=__new0  BranchType=RL  Resistance=R_7_8  Inductance=L_7_8  SetiL0=off  InitialCurrent=0  Capacitance=1e-6  Setx0=off  InitialVoltage=0  Measurements=None
  2 : powerlib/Elements/Series RLC Branch  LConnTagsString=__new0  RConnTagsString=__new0  BranchType=RL  Resistance=R_7_8  Inductance=L_7_8  SetiL0=off  InitialCurrent=0  Capacitance=1e-6  Setx0=off  InitialVoltage=0  Measurements=None
  3 : powerlib/Elements/Series RLC Branch  LConnTagsString=__new0  RConnTagsString=__new0  BranchType=RL  Resistance=R_7_8  Inductance=L_7_8  SetiL0=off  InitialCurrent=0  Capacitance=1e-6  Setx0=off  InitialVoltage=0  Measurements=None
  A : PMIOPort  Port=1  Side=Left
  a : PMIOPort  Port=2  Side=Right
  B : PMIOPort  Port=3  Side=Left
  b : PMIOPort  Port=4  Side=Right
  C : PMIOPort  Port=5  Side=Left
  c : PMIOPort  Port=6  Side=Right
  connections:
  1/LConn1 -- A/RConn1
  2/LConn1 -- B/RConn1
  3/LConn1 -- C/RConn1
  1/RConn1 -- a/RConn1
  2/RConn1 -- b/RConn1
  3/RConn1 -- c/RConn1

== system MR_CIGRE_CONVENCIONAL/R8_R9 ==
  1 : powerlib/Elements/Series RLC Branch  LConnTagsString=__new0  RConnTagsString=__new0  BranchType=RL  Resistance=R_8_9  Inductance=L_8_9  SetiL0=off  InitialCurrent=0  Capacitance=1e-6  Setx0=off  InitialVoltage=0  Measurements=None
  2 : powerlib/Elements/Series RLC Branch  LConnTagsString=__new0  RConnTagsString=__new0  BranchType=RL  Resistance=R_8_9  Inductance=L_8_9  SetiL0=off  InitialCurrent=0  Capacitance=1e-6  Setx0=off  InitialVoltage=0  Measurements=None
  3 : powerlib/Elements/Series RLC Branch  LConnTagsString=__new0  RConnTagsString=__new0  BranchType=RL  Resistance=R_8_9  Inductance=L_8_9  SetiL0=off  InitialCurrent=0  Capacitance=1e-6  Setx0=off  InitialVoltage=0  Measurements=None
  A : PMIOPort  Port=1  Side=Left
  a : PMIOPort  Port=2  Side=Right
  B : PMIOPort  Port=3  Side=Left
  b : PMIOPort  Port=4  Side=Right
  C : PMIOPort  Port=5  Side=Left
  c : PMIOPort  Port=6  Side=Right
  connections:
  1/LConn1 -- A/RConn1
  2/LConn1 -- B/RConn1
  3/LConn1 -- C/RConn1
  1/RConn1 -- a/RConn1
  2/RConn1 -- b/RConn1
  3/RConn1 -- c/RConn1

== system MR_CIGRE_CONVENCIONAL/R9_R10 ==
  1 : powerlib/Elements/Series RLC Branch  LConnTagsString=__new0  RConnTagsString=__new0  BranchType=RL  Resistance=R_9_10  Inductance=L_9_10  SetiL0=off  InitialCurrent=0  Capacitance=1e-6  Setx0=off  InitialVoltage=0  Measurements=None
  2 : powerlib/Elements/Series RLC Branch  LConnTagsString=__new0  RConnTagsString=__new0  BranchType=RL  Resistance=R_9_10  Inductance=L_9_10  SetiL0=off  InitialCurrent=0  Capacitance=1e-6  Setx0=off  InitialVoltage=0  Measurements=None
  3 : powerlib/Elements/Series RLC Branch  LConnTagsString=__new0  RConnTagsString=__new0  BranchType=RL  Resistance=R_9_10  Inductance=L_9_10  SetiL0=off  InitialCurrent=0  Capacitance=1e-6  Setx0=off  InitialVoltage=0  Measurements=None
  A : PMIOPort  Port=1  Side=Left
  a : PMIOPort  Port=2  Side=Right
  B : PMIOPort  Port=3  Side=Left
  b : PMIOPort  Port=4  Side=Right
  C : PMIOPort  Port=5  Side=Left
  c : PMIOPort  Port=6  Side=Right
  connections:
  1/LConn1 -- A/RConn1
  2/LConn1 -- B/RConn1
  3/LConn1 -- C/RConn1
  1/RConn1 -- a/RConn1
  2/RConn1 -- b/RConn1
  3/RConn1 -- c/RConn1

== system MR_CIGRE_CONVENCIONAL/R9_R17 ==
  1 : powerlib/Elements/Series RLC Branch  LConnTagsString=__new0  RConnTagsString=__new0  BranchType=RL  Resistance=R_9_17  Inductance=L_9_17  SetiL0=off  InitialCurrent=0  Capacitance=1e-6  Setx0=off  InitialVoltage=0  Measurements=None
  2 : powerlib/Elements/Series RLC Branch  LConnTagsString=__new0  RConnTagsString=__new0  BranchType=RL  Resistance=R_9_17  Inductance=L_9_17  SetiL0=off  InitialCurrent=0  Capacitance=1e-6  Setx0=off  InitialVoltage=0  Measurements=None
  3 : powerlib/Elements/Series RLC Branch  LConnTagsString=__new0  RConnTagsString=__new0  BranchType=RL  Resistance=R_9_17  Inductance=L_9_17  SetiL0=off  InitialCurrent=0  Capacitance=1e-6  Setx0=off  InitialVoltage=0  Measurements=None
  A : PMIOPort  Port=1  Side=Left
  a : PMIOPort  Port=2  Side=Right
  B : PMIOPort  Port=3  Side=Left
  b : PMIOPort  Port=4  Side=Right
  C : PMIOPort  Port=5  Side=Left
  c : PMIOPort  Port=6  Side=Right
  connections:
  1/LConn1 -- A/RConn1
  2/LConn1 -- B/RConn1
  3/LConn1 -- C/RConn1
  1/RConn1 -- a/RConn1
  2/RConn1 -- b/RConn1
  3/RConn1 -- c/RConn1

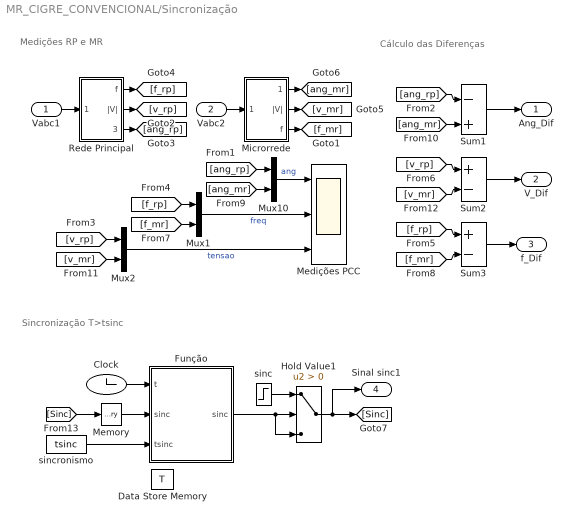
== system MR_CIGRE_CONVENCIONAL/Sincronização ==
  note: Cálculo das Diferenças
  note: Medições RP e MR
  note: Sincronização T>tsinc
  Vabc1 : Inport
  Vabc2 : Inport  Port=2
  Clock : Clock
  Data Store Memory : DataStoreMemory  DataStoreName=T  ReadBeforeWriteMsg=warning  WriteAfterWriteMsg=warning  WriteAfterReadMsg=warning  ShowAdditionalParam=off  OutDataTypeStr=double
  Função : MATLAB Function  TreatAsAtomicUnit=on
  Hold Value1 : Switch  Criteria=u2 > Threshold
  Medições PCC : Scope  NumInputPorts=3
  Memory : Memory
  Microrrede : Subsystem
  Mux1 : Mux  Inputs=2
  Mux10 : Mux  Inputs=2
  Mux2 : Mux  Inputs=2
  Rede Principal : Subsystem
  Sum1 : Sum  Inputs=-|+
  Sum2 : Sum  Inputs=+|-
  Sum3 : Sum  Inputs=+|-
  "sinc " : Step  Time=0  Before=1  SampleTime=0
  sincronismo : Constant  Value=tsinc
  Ang_Dif : Outport
  V_Dif : Outport  Port=2
  f_Dif : Outport  Port=3
  Sinal sinc1 : Outport  Port=4
  wires:
  Vabc1/1 -> Rede Principal/1(Vabc)
  Sum1/1 -> Ang_Dif/1
  Sum2/1 -> V_Dif/1
  Sum3/1 -> f_Dif/1
  Vabc2/1 -> Microrrede/1(Vabc)
  Rede Principal/1(f) -> [f_rp]
  Rede Principal/2(|V|) -> [v_rp]
  Rede Principal/3(Ang) -> [ang_rp]
  [f_rp] -> Sum3/1
  Microrrede/3(f) -> [f_mr]
  Microrrede/2(|V|) -> [v_mr]
  Microrrede/1(Ang) -> [ang_mr]
  [ang_mr] -> Sum1/2
  [ang_rp] -> Sum1/1
  [ang_mr] -> Mux10/2
  [ang_rp] -> Mux10/1
  Mux10/1 -> Medições PCC/1  "ang"
  Mux1/1 -> Medições PCC/2  "freq"
  [f_rp] -> Mux1/1
  [f_mr] -> Mux1/2
  [v_rp] -> Mux2/1
  [v_mr] -> Mux2/2
  [f_mr] -> Sum3/2
  [v_rp] -> Sum2/1
  [v_mr] -> Sum2/2
  Mux2/1 -> Medições PCC/3  "tensao"
  sincronismo/1 -> Função/3(tsinc)
  Hold Value1/1 -> [Sinc], Sinal sinc1/1
  Clock/1 -> Função/1(t)
  "sinc "/1 -> Hold Value1/1
  Memory/1 -> Função/2("sinc ")
  [Sinc] -> Memory/1
  Função/1(sinc) -> Hold Value1/3, Hold Value1/2

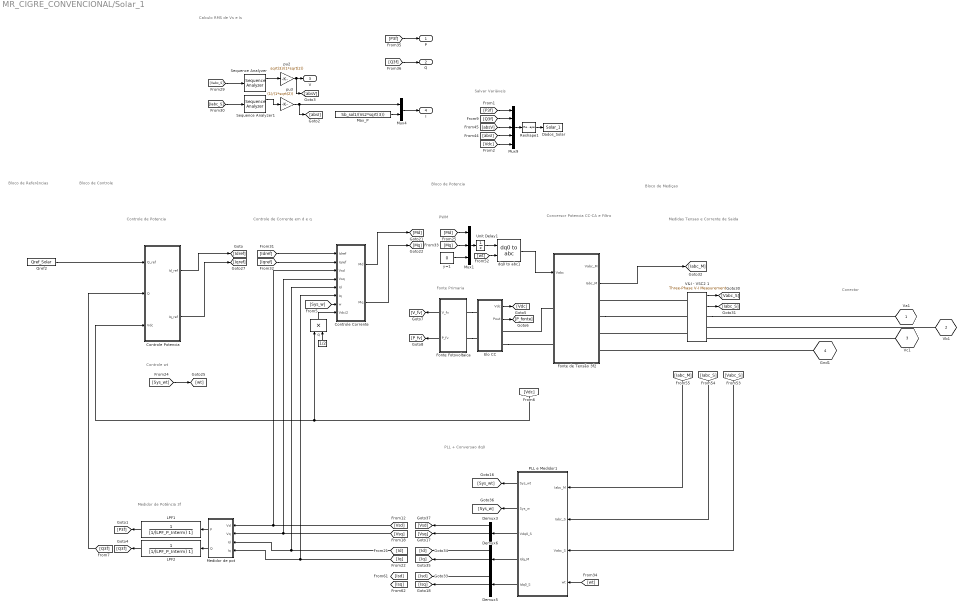
== system MR_CIGRE_CONVENCIONAL/Solar_1 ==
  note: Bloco de Controle
  note: Controle de Corrente
      |      em d e q
  note: Calculo RMS de Vs e Is
  note: Medidor de Potência 3f
  note: PWM
  note: Conversor Potencia
      |     CC-CA e Filtro
  note: Bloco de Potencia
  note: Bloco de Mediçao
  note: Medidas Tensao e
      |    Corrente de Saida
  note: PLL + Conversao dq0
  note: Controle wt
  note: Conector
  note: Salvar Variáveis
  note: Controle de
      |   Potencia
  note: Bloco de
      | Referências
  note: Fonte Primaria
  " " : Constant  Value=1/2
  Controle Corrente : Subsystem
  "Controle Potencia " : Subsystem
  Dados_Solar : ToWorkspace  VariableName=Solar_1  SaveFormat=Structure With Time  SampleTime=-1
  Demux3 : Demux  Outputs=3
  Demux5 : Demux  Outputs=3
  Demux6 : Demux  Outputs=3
  Elo CC : Subsystem
  Fonte Fotovoltaica : Subsystem
  Fonte de Tensão 3f2 : Subsystem
  LPF1 : TransferFcn  Denominator=[1/(LPF_P_Interm) 1]
  LPF2 : TransferFcn  Denominator=[1/(LPF_P_Interm) 1]
  Max_P : Constant  Value=Sb_sol1/(Vs2*sqrt(3))
  Medidor de pot : Subsystem
  Mux1 : Mux  Inputs=3
  Mux4 : Mux  Inputs=2
  Mux9 : Mux  Inputs=5
  PLL e Medidor1 : Subsystem
  Qref2 : Constant  Value=Qref_Solar
  Reshape1 : Reshape  OutputDimensions=[1,7]
  Sequence Analyzer : powerlib_meascontrol/Measurements/Sequence Analyzer  Freq=f0  n=1  seq=Positive  InInit=[1, 0]  Ts=0
      settings: SourceProductName=Simscape Power Systems  SourceProductBaseCode=PS
  Sequence Analyzer1 : powerlib_meascontrol/Measurements/Sequence Analyzer  Freq=f0  n=1  seq=Positive  InInit=[1, 0]  Ts=0
      settings: SourceProductName=Simscape Power Systems  SourceProductBaseCode=PS
  Unit Delay1 : UnitDelay  SampleTime=5E-5
  V&I - VSC2 1 : powerlib/Measurements/Three-Phase V-I Measurement  VoltageMeasurement=phase-to-ground  SetLabelV=off  LabelV=Vabc  Vpu=off  VpuLL=off  CurrentMeasurement=yes  SetLabelI=off  LabelI=Iabc  Ipu=off  Pbase=100e6  Vbase=500e3  OutputType=Complex  PhasorSimulation=off  PSBequivalent=0
  dq0 to abc1 : powerlib_meascontrol/Transformations/dq0 to abc  Alignment=90 degrees behind phase A axis
  pu2 : Gain  Gain=sqrt(3)/(1*sqrt(2))
  pu3 : Gain  Gain=(1)/(1*sqrt(2))
  q : Product  Inputs=**
  y=1 : Constant  Value=0
  Va1 : PMIOPort  Port=1  Side=Right
  Vb1 : PMIOPort  Port=2  Side=Right
  Vc1 : PMIOPort  Port=3  Side=Right
  Gnd1 : PMIOPort  Port=4  Side=Left
  P : Outport
  Q : Outport  Port=2
  V : Outport  Port=3
  I : Outport  Port=4
  wires:
  Sequence Analyzer/1 -> pu2/1
  pu2/1 -> [absV], V/1
  Sequence Analyzer1/1 -> pu3/1
  [Vabc_S] -> Sequence Analyzer/1
  [Iabc_S] -> Sequence Analyzer1/1
  [Sys_w] -> Controle Corrente/7(w)
  [Id] -> Controle Corrente/5(Id), Medidor de pot/3(Id)
  [Iq] -> Medidor de pot/4(Iq), Controle Corrente/6(Iq)
  [Idref] -> Controle Corrente/1(Idref)
  [Iqref] -> Controle Corrente/2(Iqref)
  Mux4/1 -> I/1
  pu3/1 -> Mux4/1, [absI]
  Controle Corrente/2(Mq) -> [Mq]
  q/1 -> Controle Corrente/8(Vdc/2)
  [Q3f] -> Q/1
  Max_P/1 -> Mux4/2
  "Controle Potencia "/1(Id_ref) -> [Idref]
  "Controle Potencia "/2(Iq_ref) -> [Iqref]
  [Mq] -> Mux1/2
  [Md] -> Mux1/1
  V&I - VSC2 1/2 -> [Iabc_S]
  V&I - VSC2 1/1 -> [Vabc_S]
  [wt] -> dq0 to abc1/2
  Mux1/1 -> Unit Delay1/1
  dq0 to abc1/1 -> Fonte de Tensão 3f2/1(Vabc)
  Unit Delay1/1 -> dq0 to abc1/1
  y=1/1 -> Mux1/3
  Fonte de Tensão 3f2/2(Iabc_M) -> [Iabc_M]
  Demux6/1 -> [Id]
  [wt] -> PLL e Medidor1/4(wt)
  PLL e Medidor1/5(Idq0_S) -> Demux5/1
  [Iabc_S] -> PLL e Medidor1/2(Iabc_S)
  PLL e Medidor1/4(Idq_M) -> Demux6/1
  PLL e Medidor1/3(Vdq0_S) -> Demux3/1
  [Vabc_S] -> PLL e Medidor1/3(Vabc_S)
  [Iabc_M] -> PLL e Medidor1/1(Iabc_M)
  Demux5/1 -> [Isd]
  Demux6/2 -> [Iq]
  PLL e Medidor1/2(Sys_w) -> [Sys_w]
  Demux3/1 -> [Vsd]
  PLL e Medidor1/1(Sys_wt) -> [Sys_wt]
  Demux5/2 -> [Isq]
  Demux3/2 -> [Vsq]
  [Vsd] -> Controle Corrente/3(Vsd), Medidor de pot/1(Vd)
  [Vsq] -> Medidor de pot/2(Vq), Controle Corrente/4(Vsq)
  [P3f] -> P/1
  [Sys_wt] -> [wt]
  Reshape1/1 -> Dados_Solar/1
  [P3f] -> Mux9/1
  [absV] -> Mux9/3
  Mux9/1 -> Reshape1/1
  [Q3f] -> Mux9/2
  [absI] -> Mux9/4
  Medidor de pot/2(Q) -> LPF2/1
  LPF1/1 -> [P3f]
  LPF2/1 -> [Q3f]
  Medidor de pot/1(P) -> LPF1/1
  Elo CC/1(Vdc) -> [Vdc]
  Elo CC/2(Pout) -> [P_fonte]
  Fonte Fotovoltaica/1(V_fv) -> [V_fv]
  Fonte Fotovoltaica/2(P_fv) -> [P_fv]
  [Q3f] -> "Controle Potencia "/2(Q)
  Qref2/1 -> "Controle Potencia "/1(Q_ref)
  Controle Corrente/1(Md) -> [Md]
  " "/1 -> q/2
  [Vdc] -> q/1, "Controle Potencia "/3(Vdc)
  [Vdc] -> Mux9/5
  connections:
  Gnd1/RConn1 -- Fonte de Tensão 3f2/RConn4
  Fonte de Tensão 3f2/RConn2 -- V&I - VSC2 1/LConn2
  V&I - VSC2 1/RConn1 -- Va1/RConn1
  V&I - VSC2 1/LConn1 -- Fonte de Tensão 3f2/RConn1
  V&I - VSC2 1/LConn3 -- Fonte de Tensão 3f2/RConn3
  Vb1/RConn1 -- V&I - VSC2 1/RConn2
  Vc1/RConn1 -- V&I - VSC2 1/RConn3
  Elo CC/RConn2 -- Fonte de Tensão 3f2/LConn2
  Fonte de Tensão 3f2/LConn1 -- Elo CC/RConn1
  Fonte Fotovoltaica/LConn1 -- Elo CC/LConn1
  Fonte Fotovoltaica/LConn2 -- Elo CC/LConn2

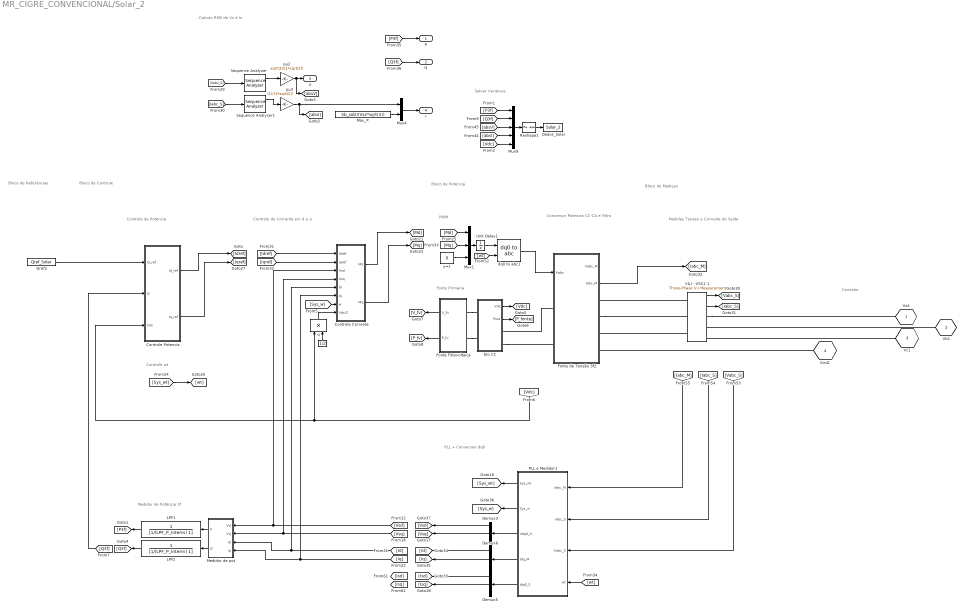
== system MR_CIGRE_CONVENCIONAL/Solar_2 ==
  note: Bloco de Controle
  note: Controle de Corrente
      |      em d e q
  note: Calculo RMS de Vs e Is
  note: Medidor de Potência 3f
  note: PWM
  note: Conversor Potencia
      |     CC-CA e Filtro
  note: Bloco de Potencia
  note: Bloco de Mediçao
  note: Medidas Tensao e
      |    Corrente de Saida
  note: PLL + Conversao dq0
  note: Controle wt
  note: Conector
  note: Salvar Variáveis
  note: Controle de
      |   Potencia
  note: Bloco de
      | Referências
  note: Fonte Primaria
  " " : Constant  Value=1/2
  Controle Corrente : Subsystem
  "Controle Potencia " : Subsystem
  Dados_Solar : ToWorkspace  VariableName=Solar_2  SaveFormat=Structure With Time  SampleTime=-1
  Demux3 : Demux  Outputs=3
  Demux5 : Demux  Outputs=3
  Demux6 : Demux  Outputs=3
  Elo CC : Subsystem
  Fonte Fotovoltaica : Subsystem
  Fonte de Tensão 3f2 : Subsystem
  LPF1 : TransferFcn  Denominator=[1/(LPF_P_Interm) 1]
  LPF2 : TransferFcn  Denominator=[1/(LPF_P_Interm) 1]
  Max_P : Constant  Value=Sb_sol2/(Vs2*sqrt(3))
  Medidor de pot : Subsystem
  Mux1 : Mux  Inputs=3
  Mux4 : Mux  Inputs=2
  Mux9 : Mux  Inputs=5
  PLL e Medidor1 : Subsystem
  Qref2 : Constant  Value=Qref_Solar
  Reshape1 : Reshape  OutputDimensions=[1,7]
  Sequence Analyzer : powerlib_meascontrol/Measurements/Sequence Analyzer  Freq=f0  n=1  seq=Positive  InInit=[1, 0]  Ts=0
      settings: SourceProductName=Simscape Power Systems  SourceProductBaseCode=PS
  Sequence Analyzer1 : powerlib_meascontrol/Measurements/Sequence Analyzer  Freq=f0  n=1  seq=Positive  InInit=[1, 0]  Ts=0
      settings: SourceProductName=Simscape Power Systems  SourceProductBaseCode=PS
  Unit Delay1 : UnitDelay  SampleTime=5E-5
  V&I - VSC2 1 : powerlib/Measurements/Three-Phase V-I Measurement  VoltageMeasurement=phase-to-ground  SetLabelV=off  LabelV=Vabc  Vpu=off  VpuLL=off  CurrentMeasurement=yes  SetLabelI=off  LabelI=Iabc  Ipu=off  Pbase=100e6  Vbase=500e3  OutputType=Complex  PhasorSimulation=off  PSBequivalent=0
  dq0 to abc1 : powerlib_meascontrol/Transformations/dq0 to abc  Alignment=90 degrees behind phase A axis
  pu2 : Gain  Gain=sqrt(3)/(1*sqrt(2))
  pu3 : Gain  Gain=(1)/(1*sqrt(2))
  q : Product  Inputs=**
  y=1 : Constant  Value=0
  Va1 : PMIOPort  Port=1  Side=Right
  Vb1 : PMIOPort  Port=2  Side=Right
  Vc1 : PMIOPort  Port=3  Side=Right
  Gnd1 : PMIOPort  Port=4  Side=Left
  P : Outport
  Q : Outport  Port=2
  V : Outport  Port=3
  I : Outport  Port=4
  wires:
  Sequence Analyzer/1 -> pu2/1
  pu2/1 -> [absV], V/1
  Sequence Analyzer1/1 -> pu3/1
  [Vabc_S] -> Sequence Analyzer/1
  [Iabc_S] -> Sequence Analyzer1/1
  [Sys_w] -> Controle Corrente/7(w)
  [Id] -> Controle Corrente/5(Id), Medidor de pot/3(Id)
  [Iq] -> Medidor de pot/4(Iq), Controle Corrente/6(Iq)
  [Idref] -> Controle Corrente/1(Idref)
  [Iqref] -> Controle Corrente/2(Iqref)
  Mux4/1 -> I/1
  pu3/1 -> Mux4/1, [absI]
  Controle Corrente/2(Mq) -> [Mq]
  q/1 -> Controle Corrente/8(Vdc/2)
  [Q3f] -> Q/1
  Max_P/1 -> Mux4/2
  "Controle Potencia "/1(Id_ref) -> [Idref]
  "Controle Potencia "/2(Iq_ref) -> [Iqref]
  [Mq] -> Mux1/2
  [Md] -> Mux1/1
  V&I - VSC2 1/2 -> [Iabc_S]
  V&I - VSC2 1/1 -> [Vabc_S]
  [wt] -> dq0 to abc1/2
  Mux1/1 -> Unit Delay1/1
  dq0 to abc1/1 -> Fonte de Tensão 3f2/1(Vabc)
  Unit Delay1/1 -> dq0 to abc1/1
  y=1/1 -> Mux1/3
  Fonte de Tensão 3f2/2(Iabc_M) -> [Iabc_M]
  Demux6/1 -> [Id]
  [wt] -> PLL e Medidor1/4(wt)
  PLL e Medidor1/5(Idq0_S) -> Demux5/1
  [Iabc_S] -> PLL e Medidor1/2(Iabc_S)
  PLL e Medidor1/4(Idq_M) -> Demux6/1
  PLL e Medidor1/3(Vdq0_S) -> Demux3/1
  [Vabc_S] -> PLL e Medidor1/3(Vabc_S)
  [Iabc_M] -> PLL e Medidor1/1(Iabc_M)
  Demux5/1 -> [Isd]
  Demux6/2 -> [Iq]
  PLL e Medidor1/2(Sys_w) -> [Sys_w]
  Demux3/1 -> [Vsd]
  PLL e Medidor1/1(Sys_wt) -> [Sys_wt]
  Demux5/2 -> [Isq]
  Demux3/2 -> [Vsq]
  [Vsd] -> Controle Corrente/3(Vsd), Medidor de pot/1(Vd)
  [Vsq] -> Medidor de pot/2(Vq), Controle Corrente/4(Vsq)
  [P3f] -> P/1
  [Sys_wt] -> [wt]
  Reshape1/1 -> Dados_Solar/1
  [P3f] -> Mux9/1
  [absV] -> Mux9/3
  Mux9/1 -> Reshape1/1
  [Q3f] -> Mux9/2
  [absI] -> Mux9/4
  Medidor de pot/2(Q) -> LPF2/1
  LPF1/1 -> [P3f]
  LPF2/1 -> [Q3f]
  Medidor de pot/1(P) -> LPF1/1
  Elo CC/1(Vdc) -> [Vdc]
  Elo CC/2(Pout) -> [P_fonte]
  Fonte Fotovoltaica/1(V_fv) -> [V_fv]
  Fonte Fotovoltaica/2(P_fv) -> [P_fv]
  [Q3f] -> "Controle Potencia "/2(Q)
  Qref2/1 -> "Controle Potencia "/1(Q_ref)
  Controle Corrente/1(Md) -> [Md]
  " "/1 -> q/2
  [Vdc] -> q/1, "Controle Potencia "/3(Vdc)
  [Vdc] -> Mux9/5
  connections:
  Gnd1/RConn1 -- Fonte de Tensão 3f2/RConn4
  Fonte de Tensão 3f2/RConn2 -- V&I - VSC2 1/LConn2
  V&I - VSC2 1/RConn1 -- Va1/RConn1
  V&I - VSC2 1/LConn1 -- Fonte de Tensão 3f2/RConn1
  V&I - VSC2 1/LConn3 -- Fonte de Tensão 3f2/RConn3
  Vb1/RConn1 -- V&I - VSC2 1/RConn2
  Vc1/RConn1 -- V&I - VSC2 1/RConn3
  Elo CC/RConn2 -- Fonte de Tensão 3f2/LConn2
  Fonte de Tensão 3f2/LConn1 -- Elo CC/RConn1
  Fonte Fotovoltaica/LConn1 -- Elo CC/LConn1
  Fonte Fotovoltaica/LConn2 -- Elo CC/LConn2

== system MR_CIGRE_CONVENCIONAL/Stop ==
  V : Inport
  f : Inport  Port=2
  P1 : Inport  Port=3
  P2 : Inport  Port=4
  P3 : Inport  Port=5
  Q1 : Inport  Port=6
  Q2 : Inport  Port=7
  Q3 : Inport  Port=8
  Modo : Inport  Port=9
  Abs : Abs
  Abs1 : Abs
  Constant : Constant
  Data Store Memory3 : DataStoreMemory  DataStoreName=C  ReadBeforeWriteMsg=warning  WriteAfterWriteMsg=warning  WriteAfterReadMsg=warning  VectorParams1D=off  ShowAdditionalParam=off  OutDataTypeStr=double
  Gain : Gain  Gain=1/Vs2
  Gain1 : Gain  Gain=1/w0
  Gain2 : Gain  Gain=1/Sb_ger
  Gain3 : Gain  Gain=1/Sb_ger
  Integrator : Integrator
  Integrator1 : Integrator
  Mux : Mux  Commented=on  Inputs=2
  Mux1 : Mux  Commented=on  Inputs=2
  Mux13 : Mux  Inputs=3
  Mux14 : Mux  Inputs=3
  Scope : Scope  Commented=on  NumInputPorts=2
  Scope1 : Scope  Commented=on  NumInputPorts=2
  Scope2 : Scope  Commented=on
  Stop Simulation : Stop
  StopSimulation : MATLAB Function  TreatAsAtomicUnit=on
  Sum : Sum  Inputs=+-|
  Sum1 : Sum  Inputs=+-|
  Sum2 : Sum  Commented=on  Inputs=+-|
  To Workspace : ToWorkspace  VariableName=STOP  SampleTime=-1
  To Workspace1 : ToWorkspace  Commented=on  VariableName=ERR  SampleTime=-1
  Transport Delay : TransportDelay  DelayTime=0.2
  Transport Delay1 : TransportDelay  DelayTime=0.3  InitialOutput=1
  wires:
  Modo/1 -> Transport Delay1/1
  StopSimulation/1(Stop) -> Stop Simulation/1, To Workspace/1
  Mux13/1 -> Gain3/1
  Mux14/1 -> Gain2/1
  P1/1 -> Mux14/1
  P2/1 -> Mux14/2
  Q3/1 -> Mux13/3
  P3/1 -> Mux14/3
  Q1/1 -> Mux13/1
  Q2/1 -> Mux13/2
  f/1 -> Gain1/1
  V/1 -> Gain/1
  Gain/1 -> StopSimulation/1(V)
  Gain1/1 -> Sum1/1, Scope1/1, Sum/1, StopSimulation/2(f)
  Gain2/1 -> StopSimulation/3(P)
  Gain3/1 -> StopSimulation/4(Q)
  Integrator1/1 -> Sum2/1, Mux/1, StopSimulation/5(Int)
  Integrator/1 -> Sum2/2, Mux/2, StopSimulation/6(IntD)
  Abs/1 -> Integrator1/1
  Abs1/1 -> Integrator/1
  Sum/1 -> Transport Delay/1
  Sum1/1 -> Mux1/1, Abs/1
  Constant/1 -> Sum/2, Sum1/2
  Mux/1 -> Scope/1
  Sum2/1 -> To Workspace1/1, Scope1/2, Scope/2
  Transport Delay/1 -> Mux1/2, Abs1/1
  Mux1/1 -> Scope2/1
  Transport Delay1/1 -> StopSimulation/7(Modo)
